simulink model "elec_inductor_hysteresis"  (R2017a)
settings: Solver=VariableStepAuto  StartTime=0.0  StopTime=4/60  MaxStep=1e-3  RelTol=1e-3  EnableMultiTasking=on
PreLoadFcn:
  | % Jiles-Atherton parameters
  | dBdH0 = 0.005;
  | B1 = 1.49;
  | H1 = 1000;
  | c = 0.1;
  | K = 200;
  | alpha = 1e-4;
  | 
  | % Vector of fractional perturbations to c, K and alpha
  | deltas = [0 0 0];
values from neighbouring files (symbols this model uses):
  Ip = (abs(clip_min)+clip_max) / 605    [extract_JA_parameters_.m]
libraries: fl_lib x3, elec_lib x1, nesl_utility x1
CloseFcn:
  | try,close(h1_elec_inductor_hysteresis),end
  | clear h1_elec_inductor_hysteresis
  | 
  | clear simlog_elec_inductor_hysteresis
  | clear logsout_elec_inductor_hysteresis
Description:
  | Inductor With Hysteresis
  | 
  | Copyright 2008-2017 The MathWorks, Inc.
settings Model: ExtModeAutoUpdateStatusClock=off  Creator=MathWorks  LastModifiedBy=Andreas
settings DataIOCC: MaxDataPoints=10000  SaveFormat=Array  SignalLoggingSaveFormat=ModelDataLogs  SignalLoggingName=logsout_elec_inductor_hysteresis
settings OptimizationCC: ExpressionDepthLimit=2147483647  InitFltsAndDblsToZero=on  EfficientMapNaN2IntZero=off  LifeSpan=inf
settings DebuggingCC: AlgebraicLoopMsg=none  UnderspecifiedInitializationDetection=Classic  MergeDetectMultiDrivingBlocksExec=none  FcnCallInpInsideContextMsg=warning  StateNameClashWarn=warning  SFUnexpectedBacktrackingDiag=warning  SFNoUnconditionalDefaultTransitionDiag=warning  SFExecutionAtInitializationDiag=none
settings HardwareCC: ProdBitPerPointer=32  ProdBitPerSizeT=32  ProdBitPerPtrDiffT=32  ProdLargestAtomicFloat=None  ProdIntDivRoundTo=Undefined  ProdEndianess=Unspecified  ProdWordSize=32  ProdHWDeviceType=32-bit Generic
settings ModelReferenceCC: PropagateSignalLabelsOutOfModel=off
settings GRTTargetCC: TargetLangStandard=C89/C90 (ANSI)  GeneratePreprocessorConditionals=Disable all  CombineOutputUpdateFcns=off  GRTInterface=on
settings ConfigComp: CovMetricSettings=dw  CovHtmlReporting=on  CovSaveCumulativeToWorkspaceVar=on  CovSaveSingleToWorkspaceVar=on  CovExternalEMLEnable=off  CovSFcnEnable=off
settings SimscapeCC: SimscapeLogType=all  SimscapeLogSimulationStatistics=on  SimscapeLogName=simlog_elec_inductor_hysteresis  SimscapeLogDataHistory=10000

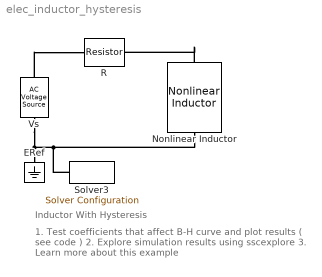
== system elec_inductor_hysteresis ==
  note: Inductor With Hysteresis
  note: 1. Test coefficients that affect B-H curve
      | and plot results ( see code )
      | 2. Explore simulation results using sscexplore
      | 3. Learn more about this example
  ERef : fl_lib/Electrical/Electrical Elements/Electrical Reference
      settings: SourceProductName=Foundation Library
  Nonlinear Inductor : elec_lib/Passive Devices/Nonlinear Inductor  parameterization_option=5  Nw=10  L=2e-4 H  L_sat=1e-4 H  current_data=[ 0 0.64 1.28 1.92 2.56 3.20 ] A  magnetic_flux_data=[0 1.29 2.00 2.27 2.36 2.39 ].*1e-5 Wb  H_data="[0   199   398   597   796   995] A/m"  B_data="[0    0.75    1.20    1.39    1.46    1.49] T"  magnetic_flux_sat=1.3e-5 Wb  length_effective=0.032 m  area_effective=1.6e-5 m^2  dBdH0=dBdH0 m*T/A  B1=B1 T  H1=H1 A/m  c=c*(1+deltas(1))  K=K*(1+deltas(2)) A/m  alpha=alpha*(1+deltas(3))  x0_option=1  i_L0=0 A  phi0=0 Wb  B0=0 T  H0=0 A/m  G_parasitic=1e-9 1/Ohm  interpolation_option=1
      settings: SourceProductName=Simscape Electronics  SourceProductBaseCode=SN
  R : fl_lib/Electrical/Electrical Elements/Resistor  R=1/Ip Ohm  i_specify=off  i_priority=High  i=0 A  i_nominal_specify=off  i_nominal_unit=A  i_nominal_value=1  v_specify=off  v_priority=High  v=0 V  v_nominal_specify=off  v_nominal_unit=V  v_nominal_value=1
      settings: SourceProductName=Foundation Library
  Solver3 : nesl_utility/Solver Configuration  PhysicalDomain=network_engine_domain  SubClassName=solver  LeftPortType=input  RightPortType=generic  Accelerate=off  Tones=[]  Harmonics=[]  SimulateNoise=off  Profile=off  UseLocalSampling=off  EnableSwitchedLinearOptims=on  FrequencyDomain=off  UseCCode=off  RelTol=0.001  AbsTol=1e-06  MinStep=1e-09  ToWorkspace=off  RevertToSquareIcSolve=off  NumHomotopyIterations=100  PhasorMode=off  PhasorModeNumHarmonics=1  OverrideAbsTol=off  DoDC=on  ResidualTolerance=1e-9  UseLocalSolver=off  LocalSolverChoice=NE_BACKWARD_EULER_ADVANCER  LocalSolverSampleTime=.0001  DoFixedCost=off  MaxNonlinIter=3  MaxModeIter=2  LinearAlgebra=Sparse  DelaysMemoryBudget=1024  AutomaticFiltering=on  FilteringTimeConstant=0.001
  Vs : fl_lib/Electrical/Electrical Sources/AC Voltage Source  amp=1 V  shift=0 deg  frequency=60 Hz  omega=0 rad/s
      settings: SourceProductName=Foundation Library
  connections:
  Nonlinear Inductor/RConn1 -- Solver3/RConn1 -- Vs/RConn1 -- ERef/LConn1
  Vs/LConn1 -- R/LConn1
  Nonlinear Inductor/LConn1 -- R/RConn1
